simulink model "demo_all"  (Simulink 7.4)
settings: Solver=ode3  StartTime=0.0  StopTime=inf  FixedStep=0.005  RelTol=1e-3
libraries: simulink x4, planmant x1, simulink_extras x1
settings Model: Creator=Admin  LastModifiedBy=Admin

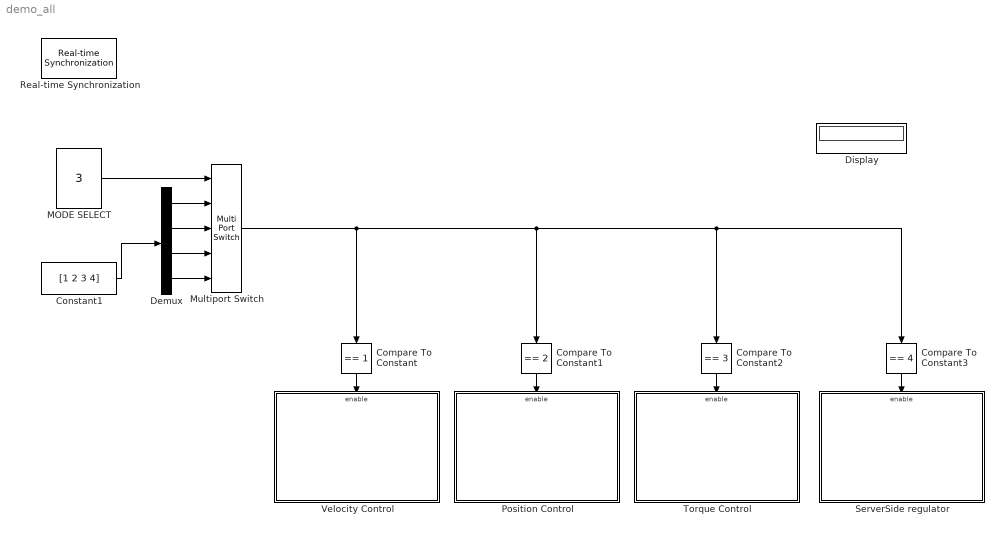
== system demo_all ==
  Compare To Constant : simulink/Logic and Bit Operations/Compare To Constant  SystemSampleTime=-1  relop===  const=1  LogicOutDataTypeMode=uint8
  Compare To Constant1 : simulink/Logic and Bit Operations/Compare To Constant  SystemSampleTime=-1  relop===  const=2  LogicOutDataTypeMode=uint8
  Compare To Constant2 : simulink/Logic and Bit Operations/Compare To Constant  SystemSampleTime=-1  relop===  const=3  LogicOutDataTypeMode=uint8
  Compare To Constant3 : simulink/Logic and Bit Operations/Compare To Constant  SystemSampleTime=-1  relop===  const=4  LogicOutDataTypeMode=uint8
  Constant1 : Constant  Value=[1 2 3 4]  OutDataType=fixdt(1, 16)  OutScaling=2^0
  Demux : Demux
  Display : Display
  MODE SELECT : Constant  Value=3  OutDataType=fixdt(1, 16)  OutScaling=2^0
  Multiport Switch : MultiPortSwitch  Inputs=4  OutDataType=fixdt(1, 16)  OutScaling=2^0
  Position Control : Subsystem
  Real-time Synchronization : planmant/Utility/Real-time Synchronization  SystemSampleTime=-1
  ServerSide regulator : Subsystem
  Torque Control : Subsystem
  Velocity Control : Subsystem
  wires:
  MODE SELECT/1 -> Multiport Switch/1
  Demux/1 -> Multiport Switch/2
  Demux/2 -> Multiport Switch/3
  Demux/3 -> Multiport Switch/4
  Demux/4 -> Multiport Switch/5
  Constant1/1 -> Demux/1
  Compare To Constant/1 -> Velocity Control/Enable
  Compare To Constant1/1 -> Position Control/Enable
  Compare To Constant2/1 -> Torque Control/Enable
  Compare To Constant3/1 -> ServerSide regulator/Enable
  Multiport Switch/1 -> Compare To Constant/1, Compare To Constant1/1, Compare To Constant2/1, Compare To Constant3/1

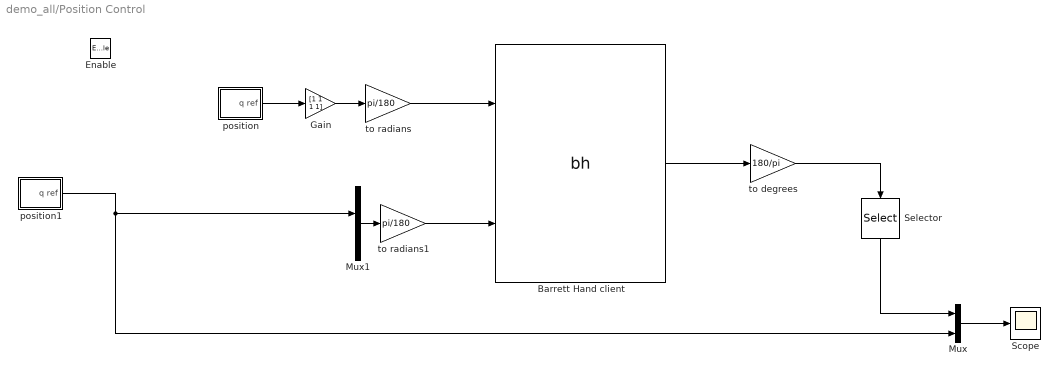
== system demo_all/Position Control ==
  Enable : EnablePort
  Barrett Hand client : S-Function  FunctionName=bh  Parameters=IP port mode262 mode280 ST a0 a1 a2 a3 a4 a41 a5 a6 a7 a8 a81 a9  EnableBusSupport=off  mask(Barrett Hand UDP client){mode262=Position, mode280=Position, IP=193.2.6.112, port=4444, ST=0.005, a0=off, a1=off, a2=off, a3=off, a4=off, a41=off, a5=on, a6=off, a7=off, a8=off, a81=off, a9=off}
      mask prompts: mode262 "BH262 mode"; mode280 "BH280 mode"; port "UDP port"; a0 "Time"; a1 "262 position"; a2 "262 velocity"; a3 "262 deltap"; a4 "262 strain"; a41 "262 strain filt"; a5 "280 position"; a6 "280 velocity"; a7 "280 deltap"; a8 "280 strain"; a81 "280 strain filt"; a9 "pps"
      mask help:
      | Make sure you select the right mode. Sending positions when velocity mode
      | selected may not end well.
      |
      | Units are rad and rad/s. Strain and pps data is raw (no units)
      mask StyleString: popup(Velocity|Position|Torque|Other),popup(Velocity|Position|Torque|Other),edit,edit,edit,checkbox,checkbox,checkbox,checkbox,checkbox,checkbox,checkbox,checkbox,checkbox,checkbox,checkbox,checkbox
      mask CallbackString: togglePorts()|togglePorts()|togglePorts()|togglePorts()||togglePorts()|togglePorts()|togglePorts()|togglePorts()|togglePorts()|togglePorts()|togglePorts()|togglePorts()|togglePorts()|togglePorts()|togglePorts()|togglePorts()
      mask TabNameString: Control,Control,Control,Control,Control,Outputs,Outputs,Outputs,Outputs,Outputs,Outputs,Outputs,Outputs,Outputs,Outputs,Outputs,Outputs
      mask Display: text(0.3, 0.9, '\fontsize{10}IP: {\bf193.2.6.112 \newline\rmport: \bf4444}', 'horizontalAlignment', 'center','texmode','on')color('blue') port_label('input',1,'\fontsize{12}BH262 {\newline\bfPosition}','texmode','on')color('blue') port_label('input',2,'\fontsize{12}BH280 {\newline\bfPosition}','texmode','on')color('black')port_label('output',1,'\fontsize{11}BH280 {\bfPosition}','texmode','on');
  Gain : Gain  Gain=[1 1 1 1]  ParameterDataType=fixdt(1, 16)  ParameterScaling=2^0  OutDataType=fixdt(1, 16)  OutScaling=2^0
  Mux : Mux  Inputs=2
  Mux1 : Mux
  Scope : Scope
      settings: YMin=40  YMax=100
  Selector : Selector  InputPortWidth=4  IndexOptions=Index vector (dialog)  Indices=2  OutputSizes=1
  position : Subsystem
  position1 : Subsystem
  to degrees : Gain  Gain=180/pi  ParameterDataType=fixdt(1, 16)  ParameterScaling=2^0  OutDataType=fixdt(1, 16)  OutScaling=2^0
  to radians : Gain  Gain=pi/180  ParameterDataType=fixdt(1, 16)  ParameterScaling=2^0  OutDataType=fixdt(1, 16)  OutScaling=2^0
  to radians1 : Gain  Gain=pi/180  ParameterDataType=fixdt(1, 16)  ParameterScaling=2^0  OutDataType=fixdt(1, 16)  OutScaling=2^0
  wires:
  Selector/1 -> Mux/1
  Mux/1 -> Scope/1
  Gain/1 -> to radians/1
  position/1(q ref) -> Gain/1
  to degrees/1 -> Selector/1
  position1/1(q ref) -> Mux/2, Mux1/2
  to radians/1 -> Barrett Hand client/1
  Barrett Hand client/1 -> to degrees/1
  to radians1/1 -> Barrett Hand client/2
  Mux1/1 -> to radians1/1

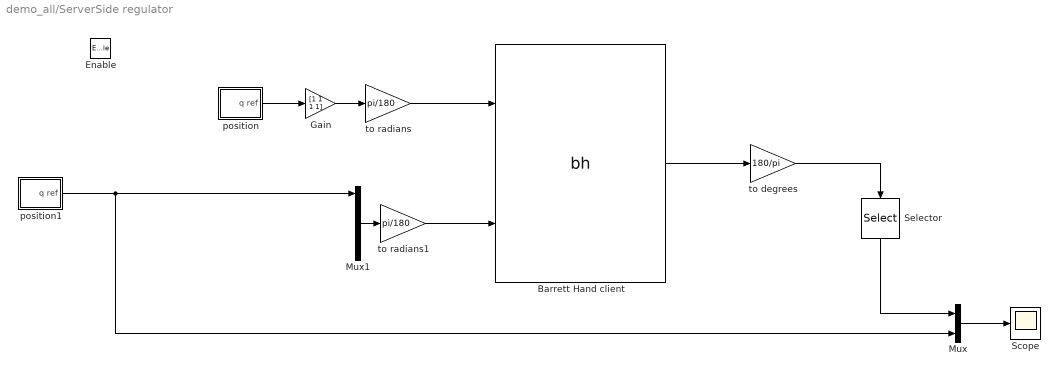
== system demo_all/ServerSide regulator ==
  Enable : EnablePort
  Barrett Hand client : S-Function  FunctionName=bh  Parameters=IP port mode262 mode280 ST a0 a1 a2 a3 a4 a41 a5 a6 a7 a8 a81 a9  EnableBusSupport=off  mask(Barrett Hand UDP client){mode262=Position, mode280=Position, IP=193.2.6.112, port=4444, ST=0.005, a0=off, a1=off, a2=off, a3=off, a4=off, a41=off, a5=on, a6=off, a7=off, a8=off, a81=off, a9=off}
      mask prompts: mode262 "BH262 mode"; mode280 "BH280 mode"; port "UDP port"; a0 "Time"; a1 "262 position"; a2 "262 velocity"; a3 "262 deltap"; a4 "262 strain"; a41 "262 strain filt"; a5 "280 position"; a6 "280 velocity"; a7 "280 deltap"; a8 "280 strain"; a81 "280 strain filt"; a9 "pps"
      mask help:
      | Make sure you select the right mode. Sending positions when velocity mode
      | selected may not end well.
      |
      | Units are rad and rad/s. Strain and pps data is raw (no units)
      mask StyleString: popup(Velocity|Position|Torque|Other),popup(Velocity|Position|Torque|Other),edit,edit,edit,checkbox,checkbox,checkbox,checkbox,checkbox,checkbox,checkbox,checkbox,checkbox,checkbox,checkbox,checkbox
      mask CallbackString: togglePorts()|togglePorts()|togglePorts()|togglePorts()||togglePorts()|togglePorts()|togglePorts()|togglePorts()|togglePorts()|togglePorts()|togglePorts()|togglePorts()|togglePorts()|togglePorts()|togglePorts()|togglePorts()
      mask TabNameString: Control,Control,Control,Control,Control,Outputs,Outputs,Outputs,Outputs,Outputs,Outputs,Outputs,Outputs,Outputs,Outputs,Outputs,Outputs
      mask Display: text(0.3, 0.9, '\fontsize{10}IP: {\bf193.2.6.112 \newline\rmport: \bf4444}', 'horizontalAlignment', 'center','texmode','on')color('blue') port_label('input',1,'\fontsize{12}BH262 {\newline\bfPosition}','texmode','on')color('blue') port_label('input',2,'\fontsize{12}BH280 {\newline\bfPosition}','texmode','on')color('black')port_label('output',1,'\fontsize{11}BH280 {\bfPosition}','texmode','on');
  Gain : Gain  Gain=[1 1 1 1]  ParameterDataType=fixdt(1, 16)  ParameterScaling=2^0  OutDataType=fixdt(1, 16)  OutScaling=2^0
  Mux : Mux  Inputs=2
  Mux1 : Mux
  Scope : Scope
      settings: YMin=40  YMax=100
  Selector : Selector  InputPortWidth=4  IndexOptions=Index vector (dialog)  Indices=1  OutputSizes=1
  position : Subsystem
  position1 : Subsystem
  to degrees : Gain  Gain=180/pi  ParameterDataType=fixdt(1, 16)  ParameterScaling=2^0  OutDataType=fixdt(1, 16)  OutScaling=2^0
  to radians : Gain  Gain=pi/180  ParameterDataType=fixdt(1, 16)  ParameterScaling=2^0  OutDataType=fixdt(1, 16)  OutScaling=2^0
  to radians1 : Gain  Gain=pi/180  ParameterDataType=fixdt(1, 16)  ParameterScaling=2^0  OutDataType=fixdt(1, 16)  OutScaling=2^0
  wires:
  Mux1/1 -> to radians1/1
  to radians1/1 -> Barrett Hand client/2
  Barrett Hand client/1 -> to degrees/1
  to radians/1 -> Barrett Hand client/1
  position1/1(q ref) -> Mux/2, Mux1/1
  to degrees/1 -> Selector/1
  position/1(q ref) -> Gain/1
  Gain/1 -> to radians/1
  Mux/1 -> Scope/1
  Selector/1 -> Mux/1

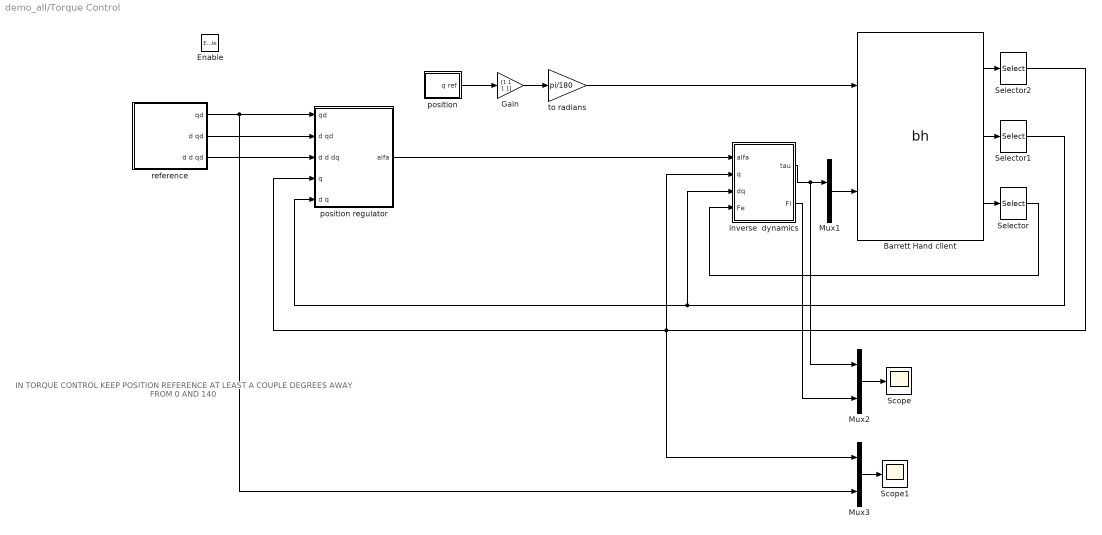
== system demo_all/Torque Control ==
  note: IN TORQUE CONTROL
      | KEEP POSITION
      | REFERENCE AT
      | LEAST A COUPLE
      | DEGREES AWAY
      | FROM 0 AND 140
  Enable : EnablePort
  Barrett Hand client : S-Function  FunctionName=bh  Parameters=IP port mode262 mode280 ST a0 a1 a2 a3 a4 a41 a5 a6 a7 a8 a81 a9  EnableBusSupport=off  mask(Barrett Hand UDP client){mode262=Torque, mode280=Torque, IP=193.2.6.112, port=4444, ST=0.005, a0=off, a1=off, a2=off, a3=off, a4=off, a41=off, a5=on, a6=on, a7=off, a8=off, a81=on, a9=off}
      mask prompts: mode262 "BH262 mode"; mode280 "BH280 mode"; port "UDP port"; a0 "Time"; a1 "262 position"; a2 "262 velocity"; a3 "262 deltap"; a4 "262 strain"; a41 "262 strain filt"; a5 "280 position"; a6 "280 velocity"; a7 "280 deltap"; a8 "280 strain"; a81 "280 strain filt"; a9 "pps"
      mask help:
      | Make sure you select the right mode. Sending positions when velocity mode
      | selected may not end well.
      |
      | Units are rad and rad/s. Strain and pps data is raw (no units)
      mask StyleString: popup(Velocity|Position|Torque|Other),popup(Velocity|Position|Torque|Other),edit,edit,edit,checkbox,checkbox,checkbox,checkbox,checkbox,checkbox,checkbox,checkbox,checkbox,checkbox,checkbox,checkbox
      mask CallbackString: togglePorts()|togglePorts()|togglePorts()|togglePorts()||togglePorts()|togglePorts()|togglePorts()|togglePorts()|togglePorts()|togglePorts()|togglePorts()|togglePorts()|togglePorts()|togglePorts()|togglePorts()|togglePorts()
      mask TabNameString: Control,Control,Control,Control,Control,Outputs,Outputs,Outputs,Outputs,Outputs,Outputs,Outputs,Outputs,Outputs,Outputs,Outputs,Outputs
      mask Display: text(0.3, 0.9, '\fontsize{10}IP: {\bf193.2.6.112 \newline\rmport: \bf4444}', 'horizontalAlignment', 'center','texmode','on')color('green') port_label('input',1,'\fontsize{12}BH262 {\newline\bfTorque}','texmode','on')color('green') port_label('input',2,'\fontsize{12}BH280 {\newline\bfTorque}','texmode','on')color('black')port_label('output',1,'\fontsize{11}BH280 {\bfPosition}','texmode','on');port_label('output',2,'BH280 {Velocity}','texmode','on');port_label('output',3,'BH280 {StrainFltr}','texmode','on');
  Gain : Gain  Gain=[1 1 1 1]  ParameterDataType=fixdt(1, 16)  ParameterScaling=2^0  OutDataType=fixdt(1, 16)  OutScaling=2^0
  Mux1 : Mux
  Mux2 : Mux  Inputs=2
  Mux3 : Mux  Inputs=2
  Scope : Scope
      settings: YMin=-400  YMax=500  SaveName=ScopeData2
  Scope1 : Scope
      settings: YMin=0.7  YMax=1.75  SaveName=ScopeData3
  Selector : Selector  InputPortWidth=4  IndexOptions=Index vector (dialog)  Indices=2  OutputSizes=1
  Selector1 : Selector  InputPortWidth=4  IndexOptions=Index vector (dialog)  Indices=2  OutputSizes=1
  Selector2 : Selector  InputPortWidth=4  IndexOptions=Index vector (dialog)  Indices=2  OutputSizes=1
  inverse  dynamics : Stateflow chart
  position : Subsystem
  position regulator : Subsystem  mask{Kp=700, Kd=100}
  reference : Subsystem
  to radians : Gain  Gain=pi/180  ParameterDataType=fixdt(1, 16)  ParameterScaling=2^0  OutDataType=fixdt(1, 16)  OutScaling=2^0
  wires:
  Gain/1 -> to radians/1
  position/1(q ref) -> Gain/1
  to radians/1 -> Barrett Hand client/1
  Mux1/1 -> Barrett Hand client/2
  inverse  dynamics/1(tau) -> Mux1/2, Mux2/1
  Barrett Hand client/2 -> Selector1/1
  Barrett Hand client/1 -> Selector2/1
  Barrett Hand client/3 -> Selector/1
  position regulator/1(alfa) -> inverse  dynamics/1(alfa)
  reference/1(qd) -> position regulator/1(qd), Mux3/2
  reference/2(d qd) -> position regulator/2(d qd)
  reference/3(d d qd) -> position regulator/3(d d dq)
  Selector/1 -> inverse  dynamics/4(Fe)
  Selector1/1 -> inverse  dynamics/3(dq), position regulator/5(d q)
  Selector2/1 -> inverse  dynamics/2(q), position regulator/4(q), Mux3/1
  Mux2/1 -> Scope/1
  inverse  dynamics/2(Fl) -> Mux2/2
  Mux3/1 -> Scope1/1

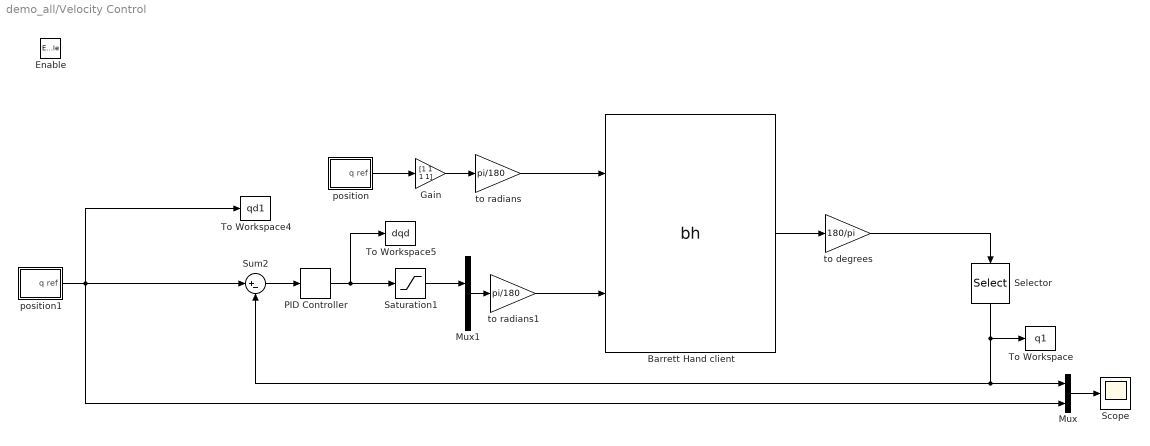
== system demo_all/Velocity Control ==
  Enable : EnablePort
  Barrett Hand client : S-Function  FunctionName=bh  Parameters=IP port mode262 mode280 ST a0 a1 a2 a3 a4 a41 a5 a6 a7 a8 a81 a9  EnableBusSupport=off  mask(Barrett Hand UDP client){mode262=Another, mode280=Velocity, IP=193.2.6.112, port=4444, ST=0.005, a0=off, a1=off, a2=off, a3=off, a4=off, a41=off, a5=on, a6=off, a7=off, a8=off, a81=off, a9=off}
      mask prompts: mode262 "BH262 mode"; mode280 "BH280 mode"; port "UDP port"; a0 "Time"; a1 "262 position"; a2 "262 velocity"; a3 "262 deltap"; a4 "262 strain"; a41 "262 strain filt"; a5 "280 position"; a6 "280 velocity"; a7 "280 deltap"; a8 "280 strain"; a81 "280 strain filt"; a9 "pps"
      mask help:
      | Make sure you select the right mode. Sending positions when velocity mode
      | selected may not end well.
      |
      | Units are rad and rad/s. Strain and pps data is raw (no units)
      mask StyleString: popup(Velocity|Position|Another),popup(Velocity|Position|Another),edit,edit,edit,checkbox,checkbox,checkbox,checkbox,checkbox,checkbox,checkbox,checkbox,checkbox,checkbox,checkbox,checkbox
      mask CallbackString: togglePorts()|togglePorts()|togglePorts()|togglePorts()||togglePorts()|togglePorts()|togglePorts()|togglePorts()|togglePorts()|togglePorts()|togglePorts()|togglePorts()|togglePorts()|togglePorts()|togglePorts()|togglePorts()
      mask TabNameString: Control,Control,Control,Control,Control,Outputs,Outputs,Outputs,Outputs,Outputs,Outputs,Outputs,Outputs,Outputs,Outputs,Outputs,Outputs
      mask Display: text(0.3, 0.9, '\fontsize{10}IP: {\bf193.2.6.112 \newline\rmport: \bf4444}', 'horizontalAlignment', 'center','texmode','on')color('black') port_label('input',1,'\fontsize{12}BH262 {\newline\bfTorque}','texmode','on')color('red') port_label('input',2,'\fontsize{12}BH280  {\newline\bfVelocity}','texmode','on')color('black')port_label('output',1,'\fontsize{11}BH280 {\bfPosition}','texmode','on');
  Gain : Gain  Gain=[1 1 1 1]  ParameterDataType=fixdt(1, 16)  ParameterScaling=2^0  OutDataType=fixdt(1, 16)  OutScaling=2^0
  Mux : Mux  Inputs=2
  Mux1 : Mux
  PID Controller : simulink_extras/Additional Linear/PID Controller  SystemSampleTime=-1  P=0.006  I=0  D=0
  Saturation1 : Saturate  UpperLimit=0.1  LowerLimit=-0.1  OutDataType=fixdt(1, 16)  OutScaling=2^0
  Scope : Scope
      settings: YMin=0  YMax=14
  Selector : Selector  InputPortWidth=4  IndexOptions=Index vector (dialog)  Indices=2  OutputSizes=1
  Sum2 : Sum  Inputs=|+-  OutDataType=fixdt(1, 16)  OutScaling=2^0
  To Workspace : ToWorkspace  VariableName=q1  SampleTime=-1  SaveFormat=Structure
  To Workspace4 : ToWorkspace  VariableName=qd1  SampleTime=-1  SaveFormat=Structure With Time
  To Workspace5 : ToWorkspace  VariableName=dqd  SampleTime=-1  SaveFormat=Structure
  position : Subsystem
  position1 : Subsystem
  to degrees : Gain  Gain=180/pi  ParameterDataType=fixdt(1, 16)  ParameterScaling=2^0  OutDataType=fixdt(1, 16)  OutScaling=2^0
  to radians : Gain  Gain=pi/180  ParameterDataType=fixdt(1, 16)  ParameterScaling=2^0  OutDataType=fixdt(1, 16)  OutScaling=2^0
  to radians1 : Gain  Gain=pi/180  ParameterDataType=fixdt(1, 16)  ParameterScaling=2^0  OutDataType=fixdt(1, 16)  OutScaling=2^0
  wires:
  Selector/1 -> To Workspace/1, Mux/1, Sum2/2
  Gain/1 -> to radians/1
  position/1(q ref) -> Gain/1
  Mux1/1 -> to radians1/1
  to degrees/1 -> Selector/1
  position1/1(q ref) -> To Workspace4/1, Mux/2, Sum2/1
  to radians/1 -> Barrett Hand client/1
  PID Controller/1 -> To Workspace5/1, Saturation1/1
  Sum2/1 -> PID Controller/1
  to radians1/1 -> Barrett Hand client/2
  Saturation1/1 -> Mux1/2
  Mux/1 -> Scope/1
  Barrett Hand client/1 -> to degrees/1

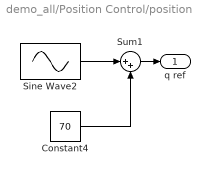
== system demo_all/Position Control/position ==
  Constant4 : Constant  Value=70  OutDataType=fixdt(1, 16)  OutScaling=2^0
  Sine Wave2 : Sin  Amplitude=30  Bias=0  Frequency=pi  Phase=pi/4  Samples=10  Offset=0
  Sum1 : Sum  Inputs=|++  OutDataType=fixdt(1, 16)  OutScaling=2^0
  q ref : Outport
  wires:
  Sum1/1 -> q ref/1
  Constant4/1 -> Sum1/2
  Sine Wave2/1 -> Sum1/1

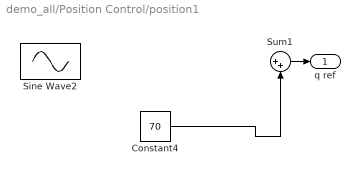
== system demo_all/Position Control/position1 ==
  Constant4 : Constant  Value=70  OutDataType=fixdt(1, 16)  OutScaling=2^0
  Sine Wave2 : Sin  Amplitude=30  Bias=0  Frequency=0.5*pi  Phase=pi/4  Samples=10  Offset=0
  Sum1 : Sum  Inputs=|++  OutDataType=fixdt(1, 16)  OutScaling=2^0
  q ref : Outport
  wires:
  Sum1/1 -> q ref/1
  Constant4/1 -> Sum1/2

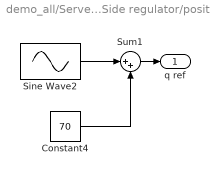
== system demo_all/ServerSide regulator/position ==
  Constant4 : Constant  Value=70  OutDataType=fixdt(1, 16)  OutScaling=2^0
  Sine Wave2 : Sin  Amplitude=30  Bias=0  Frequency=pi  Phase=pi/4  Samples=10  Offset=0
  Sum1 : Sum  Inputs=|++  OutDataType=fixdt(1, 16)  OutScaling=2^0
  q ref : Outport
  wires:
  Sine Wave2/1 -> Sum1/1
  Constant4/1 -> Sum1/2
  Sum1/1 -> q ref/1

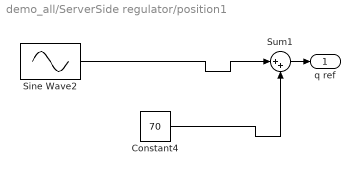
== system demo_all/ServerSide regulator/position1 ==
  Constant4 : Constant  Value=70  OutDataType=fixdt(1, 16)  OutScaling=2^0
  Sine Wave2 : Sin  Amplitude=30  Bias=0  Frequency=0.5*pi  Phase=pi/4  Samples=10  Offset=0
  Sum1 : Sum  Inputs=|++  OutDataType=fixdt(1, 16)  OutScaling=2^0
  q ref : Outport
  wires:
  Sine Wave2/1 -> Sum1/1
  Constant4/1 -> Sum1/2
  Sum1/1 -> q ref/1

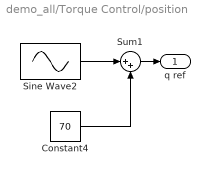
== system demo_all/Torque Control/position ==
  Constant4 : Constant  Value=70  OutDataType=fixdt(1, 16)  OutScaling=2^0
  Sine Wave2 : Sin  Amplitude=30  Bias=0  Frequency=pi  Phase=pi/4  Samples=10  Offset=0
  Sum1 : Sum  Inputs=|++  OutDataType=fixdt(1, 16)  OutScaling=2^0
  q ref : Outport
  wires:
  Sum1/1 -> q ref/1
  Constant4/1 -> Sum1/2
  Sine Wave2/1 -> Sum1/1

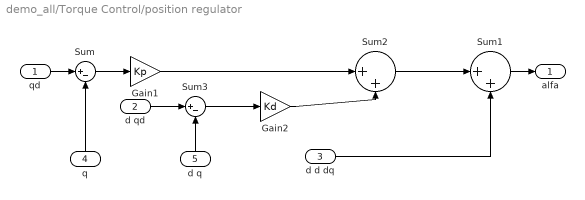
== system demo_all/Torque Control/position regulator ==
  qd : Inport
  d qd : Inport  Port=2
  d d dq : Inport  Port=3
  q : Inport  Port=4
  d q : Inport  Port=5
  Gain1 : Gain  Gain=Kp  ParameterDataType=fixdt(1, 16)  ParameterScaling=2^0  OutDataType=fixdt(1, 16)  OutScaling=2^0
  Gain2 : Gain  Gain=Kd  ParameterDataType=fixdt(1, 16)  ParameterScaling=2^0  OutDataType=fixdt(1, 16)  OutScaling=2^0
  Sum : Sum  Inputs=|+-  OutDataType=fixdt(1, 16)  OutScaling=2^0
  Sum1 : Sum  Inputs=|++  OutDataType=fixdt(1, 16)  OutScaling=2^0
  Sum2 : Sum  Inputs=|++  OutDataType=fixdt(1, 16)  OutScaling=2^0
  Sum3 : Sum  Inputs=|+-  OutDataType=fixdt(1, 16)  OutScaling=2^0
  alfa : Outport
  wires:
  Sum/1 -> Gain1/1
  Sum3/1 -> Gain2/1
  Gain1/1 -> Sum2/1
  Gain2/1 -> Sum2/2
  Sum2/1 -> Sum1/1
  q/1 -> Sum/2
  d q/1 -> Sum3/2
  qd/1 -> Sum/1
  Sum1/1 -> alfa/1
  d d dq/1 -> Sum1/2
  d qd/1 -> Sum3/1

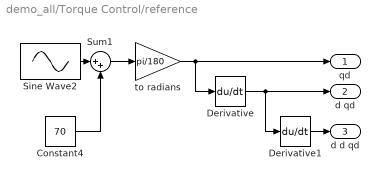
== system demo_all/Torque Control/reference ==
  Constant4 : Constant  Value=70  OutDataType=fixdt(1, 16)  OutScaling=2^0
  Derivative : Derivative
  Derivative1 : Derivative
  Sine Wave2 : Sin  Amplitude=30  Bias=0  Frequency=0.5*pi  Phase=pi/4  Samples=10  Offset=0
  Sum1 : Sum  Inputs=|++  OutDataType=fixdt(1, 16)  OutScaling=2^0
  to radians : Gain  Gain=pi/180  ParameterDataType=fixdt(1, 16)  ParameterScaling=2^0  OutDataType=fixdt(1, 16)  OutScaling=2^0
  qd : Outport
  d qd : Outport  Port=2
  d d qd : Outport  Port=3
  wires:
  Sum1/1 -> to radians/1
  Constant4/1 -> Sum1/2
  Sine Wave2/1 -> Sum1/1
  Derivative/1 -> d qd/1, Derivative1/1
  Derivative1/1 -> d d qd/1
  to radians/1 -> qd/1, Derivative/1

== system demo_all/Velocity Control/position ==
  Constant4 : Constant  Value=70  OutDataType=fixdt(1, 16)  OutScaling=2^0
  Sine Wave2 : Sin  Amplitude=30  Bias=0  Frequency=pi  Phase=pi/4  Samples=10  Offset=0
  Sum1 : Sum  Inputs=|++  OutDataType=fixdt(1, 16)  OutScaling=2^0
  q ref : Outport
  wires:
  Sum1/1 -> q ref/1
  Constant4/1 -> Sum1/2
  Sine Wave2/1 -> Sum1/1

== system demo_all/Velocity Control/position1 ==
  Constant4 : Constant  Value=70  OutDataType=fixdt(1, 16)  OutScaling=2^0
  Sine Wave2 : Sin  Amplitude=30  Bias=0  Frequency=0.5*pi  Phase=pi/4  Samples=10  Offset=0
  Sum1 : Sum  Inputs=|++  OutDataType=fixdt(1, 16)  OutScaling=2^0
  q ref : Outport
  wires:
  Sum1/1 -> q ref/1
  Constant4/1 -> Sum1/2
  Sine Wave2/1 -> Sum1/1

== matlab function Torque Control/inverse dynamics ==
  data: alfa input double; q input double; dq input double; Fe input double; tau output double; Fl output double
function [tau,Fl] = fcn(alfa,q,dq,Fe)
%#eml
B_q=1;
C_q_dq=0;
F=0.1;
Fl=300*StaticFrictionKoef(dq,alfa);
g_q=0;
Kfe=0;

tau=B_q * alfa + ...    % inertia
    C_q_dq * dq + ...   % coriollis
    F * dq + ...        % friction 
    Fl  + ...           % static friction
    g_q +...            % gravity
    Kfe * Fe;                 % environment

function Fl=StaticFrictionKoef(dq,alfa)
sig=0.4;
KFl=1;

gauss=1/(sig*sqrt(2*pi))*exp(-4*(dq/sig).^2);

Fl=KFl*gauss*sign(alfa);
